simulink model "EnergyBalancingPendulum"  (R2018b)
settings: Solver=VariableStepAuto  StartTime=0.0  StopTime=4  MaxStep=0.01  RelTol=1e-3
settings Model: Creator=Philip  LastModifiedBy=User
settings DebuggingCC: LibraryContextMissingDiagnostic=none
settings SFSimCC: SimUseLocalCustomCode=off
settings RTWCC: RTWUseLocalCustomCode=off

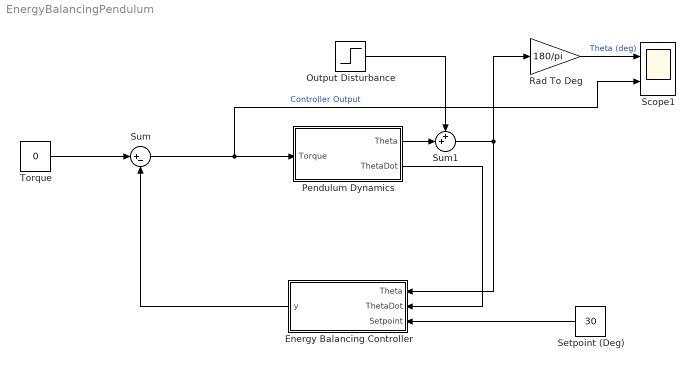
== system EnergyBalancingPendulum ==
  Energy Balancing Controller : MATLAB Function  TreatAsAtomicUnit=on
  Output Disturbance : Step  Time=2  SampleTime=0
  Pendulum Dynamics : Subsystem
  Rad To Deg : Gain  Gain=180/pi
  Scope1 : Scope  NumInputPorts=2
  Setpoint (Deg) : Constant  Value=30
  Sum : Sum  Inputs=|+-
  Sum1 : Sum  Inputs=++|
  Torque : Constant  Value=0
  wires:
  Pendulum Dynamics/2(ThetaDot) -> Energy Balancing Controller/2(ThetaDot)
  Energy Balancing Controller/1(y) -> Sum/2
  Setpoint (Deg)/1 -> Energy Balancing Controller/3(Setpoint)
  Torque/1 -> Sum/1
  Rad To Deg/1 -> Scope1/1  "Theta (deg)"
  Sum/1 -> Scope1/2, Pendulum Dynamics/1(Torque)  "Controller Output"
  Pendulum Dynamics/1(Theta) -> Sum1/2
  Sum1/1 -> Energy Balancing Controller/1(Theta), Rad To Deg/1
  Output Disturbance/1 -> Sum1/1

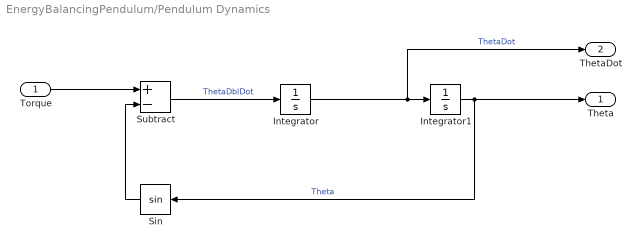
== system EnergyBalancingPendulum/Pendulum Dynamics ==
  Torque : Inport
  Integrator : Integrator
  Integrator1 : Integrator
  Sin : Trigonometry
  Subtract : Sum  Inputs=+-
  Theta : Outport
  ThetaDot : Outport  Port=2
  wires:
  Integrator1/1 -> Theta/1, Sin/1  "Theta"
  Sin/1 -> Subtract/2
  Torque/1 -> Subtract/1
  Subtract/1 -> Integrator/1  "ThetaDblDot"
  Integrator/1 -> ThetaDot/1, Integrator1/1  "ThetaDot"

== matlab function EnergyBalancingPendulum/Energy Balancing Controller ==
  data: Theta input; y output; ThetaDot input; Setpoint input
function y = fcn(Theta, ThetaDot, Setpoint)

Setpoint = Setpoint * pi / 180;

K = 1;
lambda = 0.1;
y = K/lambda * ((Theta/lambda + ThetaDot) - Setpoint/lambda);
